simulink library "HardwareIO"  (R2017b)
settings: Solver=FixedStepDiscrete  StartTime=0.0  StopTime=inf  RelTol=1e-3  EnableMultiTasking=on
undefined symbols (not defined in the file or in its folder): Normalized
libraries: dspsrcs4 x1
settings Model: Creator=mcuenant  LastModifiedBy=mcuenant
settings DataIOCC: SaveFormat=Array  SaveOutput=off  SaveTime=off
settings OptimizationCC: LifeSpan=Inf
settings DebuggingCC: SFUnexpectedBacktrackingDiag=warning  SFNoUnconditionalDefaultTransitionDiag=warning  SFExecutionAtInitializationDiag=none
settings HardwareCC: ProdBitPerPointer=32  ProdBitPerSizeT=32  ProdBitPerPtrDiffT=32  ProdLargestAtomicFloat=None  ProdWordSize=32  ProdHWDeviceType=Generic->32-bit x86 compatible
settings ModelReferenceCC: PropagateSignalLabelsOutOfModel=off
settings SFSimCC: MATLABDynamicMemAlloc=off
settings RTWCC: SystemTargetFile=ert.tlc  GenCodeOnly=on  TemplateMakefile=ert_default_tmf  GenerateReport=on  IncludeHyperlinkInReport=on  LaunchReport=on  PortableWordSizes=on  CodeProfilingSaveOptions=AllData  GenerateTraceInfo=on  GenerateTraceReport=on  GenerateTraceReportSl=on  GenerateTraceReportSf=on  GenerateTraceReportEml=on  GenerateWebview=on  GenerateCodeMetricsReport=on  GenerateCodeReplacementReport=on
settings CodeAppCC: IgnoreCustomStorageClasses=off  MaxIdLength=128  SimulinkDataObjDesc=on  SFDataObjDesc=on  InsertBlockDesc=on  StateflowObjectComments=on  MATLABSourceComments=on  ReqsInCode=on
settings ERTTargetCC: MultiwordLength=2048  GenerateSampleERTMain=on  SupportAbsoluteTime=off  SupportNonFinite=off  SupportComplex=off  ERTCustomFileTemplate=example_file_process.tlc  ConvertIfToSwitch=off  SuppressUnreachableDefaultCases=off
settings ConfigComp: CovMetricSettings=dw  CovSaveCumulativeToWorkspaceVar=on  CovSaveSingleToWorkspaceVar=on  CovExternalEMLEnable=off

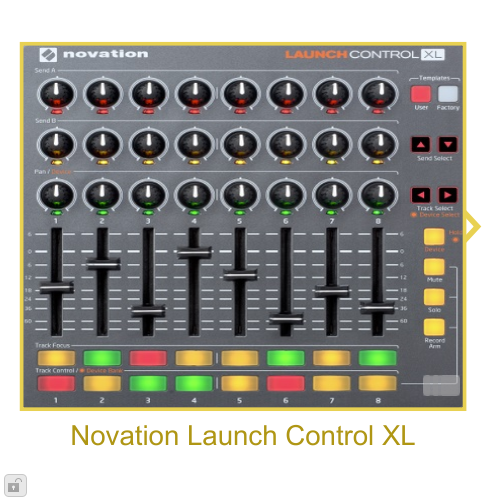
[thumbnail: Simulink's stored preview of the top-level diagram]
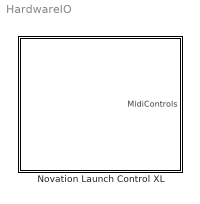
== system HardwareIO ==
  Novation Launch Control XL : Subsystem  TreatAsAtomicUnit=on  mask{Tso=0.1, Tsi=0.1, rtp=off, kA1=[0  1], kA2=[0  1], kA3=[0  1], kA4=[0  1], kA5=[0  1], kA6=[0  1], kA7=[0  1], kA8=[0  1], skA1=Linear, skA2=Linear, skA3=Linear, skA4=Linear, skA5=Linear, skA6=Linear, skA7=Linear, skA8=Linear, kB1=[0  1], kB2=[0  1], kB3=[0  1], kB4=[0  1], kB5=[0  1], kB6=[0  1], kB7=[0  1], kB8=[0  1], skB1=Linear, skB2=Linear, skB3=Linear, skB4=Linear, skB5=Linear, skB6=Linear, skB7=Linear, skB8=Linear, kC1=[0  1], kC2=[0  1], kC3=[0  1], kC4=[0  1], kC5=[0  1], kC6=[0  1], kC7=[0  1], kC8=[0  1], skC1=Linear, skC2=Linear, skC3=Linear, skC4=Linear, skC5=Linear, skC6=Linear, skC7=Linear, skC8=Linear, f1=[0  1], f2=[0  1], f3=[0  1], f4=[0  1], f5=[0  1], f6=[0  1], f7=[0  1], f8=[0  1], sf1=Linear, sf2=Linear, sf3=Linear, sf4=Linear, sf5=Linear, sf6=Linear, sf7=Linear, sf8=Linear}
      mask prompts: Tso "Output Sample Time (s)"; Tsi "Inner Sample Time for MIDI capture (s)   -   Recommended Value : 0.1 s"; rtp "Real-Time Pacer"; kA1 "Knob A1"; kA2 "Knob A2"; kA3 "Knob A3"; kA4 "Knob A4"; kA5 "Knob A5"; kA6 "Knob A6"; kA7 "Knob A7"; kA8 "Knob A8"; skA1 "Scale"; skA2 "Scale"; skA3 "Scale"; skA4 "Scale"; skA5 "Scale"; skA6 "Scale"; skA7 "Scale"; skA8 "Scale"; kB1 "Knob B1"; kB2 "Knob B2"; kB3 "Knob B3"; kB4 "Knob B4"; kB5 "Knob B5"; kB6 "Knob B6"; kB7 "Knob B7"; kB8 "Knob B8"; skB1 "Scale"; skB2 "Scale"; skB3 "Scale"; skB4 "Scale"; skB5 "Scale"; skB6 "Scale"; skB7 "Scale"; skB8 "Scale"; kC1 "Knob C1"; kC2 "Knob C2"; kC3 "Knob C3"; kC4 "Knob C4"; kC5 "Knob C5"; kC6 "Knob C6"; kC7 "Knob C7"; kC8 "Knob C8"; skC1 "Scale"; skC2 "Scale"; skC3 "Scale"; skC4 "Scale"; skC5 "Scale"; skC6 "Scale"; skC7 "Scale"; skC8 "Scale"; f1 "Fader F1"; f2 "Fader F2"; f3 "Fader F3"; f4 "Fader F4"; f5 "Fader F5"; f6 "Fader F6"; f7 "Fader F7"; f8 "Fader F8"; sf1 "Scale"; sf2 "Scale"; sf3 "Scale"; sf4 "Scale"; sf5 "Scale"; sf6 "Scale"; sf7 "Scale"; sf8 "Scale"
      mask init:
      | %% Parameters
      | maxIntervals = 20; % maximum number of values for N-ary mode
      | 
      | %% Generate cell with button names
      | knobsA = arrayfun(@(x) ['Knob A' num2str(x)],1:8,'UniformOutput',false);
      | knobsB = arrayfun(@(x) ['Knob B' num2str(x)],1:8,'UniformOutput',false);
      | knobsC = arrayfun(@(x) ['Knob C' num2str(x)],1:8,'UniformOutput',false);
      | faders = arrayfun(@(x) ['Fader F' num2str(x)],1:8,'UniformOutput',false);
      | buttons = [knobsA(:) ; knobsB(:) ; knobsC(:) ; faders(:)];
      | 
      | 
      | %% Gather parameters in an array of structures
      | param(1).value = kA1;
      | param(1).scale = skA1;
      | param(2).value = kA2;
      | param(2).scale = skA2;
      | param(3).value = kA3;
      | param(3).scale = skA3;
      | param(4).value = kA4;
      | param(4).scale = skA4;
      | param(5).value = kA5;
      | param(5).scale = skA5;
      | param(6).value = kA6;
      | param(6).scale = skA6;
      | param(7).value = kA7;
      | param(7).scale = skA7;
      | param(8).value = kA8;
      | param(8).scale = skA8;
      | param(9).value = kB1;
      | param(9).scale = skB1;
      | param(10).value = kB2;
      | param(10).scale = skB2;
      | param(11).value = kB3;
      | param(11).scale = skB3;
      | param(12).value = kB4;
      | param(12).scale = skB4;
      | param(13).value = kB5;
      | param(13).scale = skB5;
      | param(14).value = kB6;
      | param(14).scale = skB6;
      | param(15).value = kB7;
      | param(15).scale = skB7;
      | param(16).value = kB8;
      | param(16).scale = skB8;
      | param(17).value = kC1;
      | param(17).scale = skC1;
      | param(18).value = kC2;
      | param(18).scale = skC2;
      | param(19).value = kC3;
      | param(19).scale = skC3;
      | param(20).value = kC4;
      | param(20).scale = skC4;
      | param(21).value = kC5;
      | param(21).scale = skC5;
      | param(22).value = kC6;
      | param(22).scale = skC6;
      | param(23).value = kC7;
      | param(23).scale = skC7;
      | param(24).value = kC8;
      | param(24).scale = skC8;
      | param(25).value = f1;
      | param(25).scale = sf1;
      | param(26).value = f2;
      | param(26).scale = sf2;
      | param(27).value = f3;
      | param(27).scale = sf3;
      | param(28).value = f4;
      | param(28).scale = sf4;
      | param(29).value = f5;
      | param(29).scale = sf5;
      | param(30).value = f6;
      | param(30).scale = sf6;
      | param(31).value = f7;
      | param(31).scale = sf7;
      | param(32).value = f8;
      | param(32).scale = sf8;
      | 
      | %% Check User Inputs
      | funcName = 'Buttons parameters';
      | for ind=1:length(param)
      |     varName = buttons{ind};
      |     switch param(ind).scale
      |         case 1 % 'Linear'
      |             errMsgName = [varName, ' (using linear scale)'];
      |             validateattributes(param(ind).value,...
      |                 {'numeric'},{'increasing','finite','row','numel',2},...
      |                 funcName,errMsgName);
      |         case 2 % 'Logarithmic'
      |             errMsgName = [varName, ' (using log scale)'];
      |             validateattributes(param(ind).value,...
      |                 {'numeric'},{'increasing','finite','row','numel',2,'>',0},...
      |                 funcName,errMsgName);
      |         case 3 % 'Binary'
      |             errMsgName = [varName, ' (using N-ary scale)'];
      |             validateattributes(param(ind).value,...
      |                 {'numeric'},{'finite','row'},...
      |                 funcName,errMsgName);
      |             if (numel(param(ind).value) < 2 || numel(param(ind).value) > maxIntervals)
      |                 errordlg(['When using N-ary scaling, you must supply between 2 and ' num2str(maxIntervals) ' values to define intervals.'])
      |             end
      |     end
      | end
      | 
      | clear kA1 kA2 kA3 kA4 kA5 kA6 kA7 kA8 kB1 kB2 kB3 kB4 kB5 kB6 kB7 kB8 kC1 kC2 kC3 kC4 kC5 kC6 kC7 kC8 f1 f2 f3 f4 f5 f6 f7 f8 skA1 skA2 skA3 skA4 skA5 skA6 skA7 skA8 skB1 skB2 skB3 skB4 skB5 skB6 skB7 skB8 skC1 skC2 skC3 skC4 skC5 skC6 skC7 skC8 sf1 sf2 sf3 sf4 sf5 sf6 sf7 sf8;
      | clear knobsA knobsB knobsC faders buttons;
      | clear funcName varName errMsgName;
      | 
      | %% Pad with NaN to allow N-ary scale (field "value" of structure array param must have a consistent size across array elements)
      | param(1).value = [param(1).value, NaN(1,maxIntervals-length(param(1).value))];
      | param(2).value = [param(2).value, NaN(1,maxIntervals-length(param(2).value))];
      | param(3).value = [param(3).value, NaN(1,maxIntervals-length(param(3).value))];
      | param(4).value = [param(4).value, NaN(1,maxIntervals-length(param(4).value))];
      | param(5).value = [param(5).value, NaN(1,maxIntervals-length(param(5).value))];
      | param(6).value = [param(6).value, NaN(1,maxIntervals-length(param(6).value))];
      | param(7).value = [param(7).value, NaN(1,maxIntervals-length(param(7).value))];
      | param(8).value = [param(8).value, NaN(1,maxIntervals-length(param(8).value))];
      | param(9).value = [param(9).value, NaN(1,maxIntervals-length(param(9).value))];
      | param(10).value = [param(10).value, NaN(1,maxIntervals-length(param(10).value))];
      | param(11).value = [param(11).value, NaN(1,maxIntervals-length(param(11).value))];
      | param(12).value = [param(12).value, NaN(1,maxIntervals-length(param(12).value))];
      | param(13).value = [param(13).value, NaN(1,maxIntervals-length(param(13).value))];
      | param(14).value = [param(14).value, NaN(1,maxIntervals-length(param(14).value))];
      | param(15).value = [param(15).value, NaN(1,maxIntervals-length(param(15).value))];
      | param(16).value = [param(16).value, NaN(1,maxIntervals-length(param(16).value))];
      | param(17).value = [param(17).value, NaN(1,maxIntervals-length(param(17).value))];
      | param(18).value = [param(18).value, NaN(1,maxIntervals-length(param(18).value))];
      | param(19).value = [param(19).value, NaN(1,maxIntervals-length(param(19).value))];
      | param(20).value = [param(20).value, NaN(1,maxIntervals-length(param(20).value))];
      | param(21).value = [param(21).value, NaN(1,maxIntervals-length(param(21).value))];
      | param(22).value = [param(22).value, NaN(1,maxIntervals-length(param(22).value))];
      | param(23).value = [param(23).value, NaN(1,maxIntervals-length(param(23).value))];
      | param(24).value = [param(24).value, NaN(1,maxIntervals-length(param(24).value))];
      | param(25).value = [param(25).value, NaN(1,maxIntervals-length(param(25).value))];
      | param(26).value = [param(26).value, NaN(1,maxIntervals-length(param(26).value))];
      | param(27).value = [param(27).value, NaN(1,maxIntervals-length(param(27).value))];
      | param(28).value = [param(28).value, NaN(1,maxIntervals-length(param(28).value))];
      | param(29).value = [param(29).value, NaN(1,maxIntervals-length(param(29).value))];
      | param(30).value = [param(30).value, NaN(1,maxIntervals-length(param(30).value))];
      | param(31).value = [param(31).value, NaN(1,maxIntervals-length(param(31).value))];
      | param(32).value = [param(32).value, NaN(1,maxIntervals-length(param(32).value))];
      | clear maxIntervals;
      mask TypeOptions skA1: Linear | Logarithmic | N-ary
      mask TypeOptions skA2: Linear | Logarithmic | N-ary
      mask TypeOptions skA3: Linear | Logarithmic | N-ary
      mask TypeOptions skA4: Linear | Logarithmic | N-ary
      mask TypeOptions skA5: Linear | Logarithmic | N-ary
      mask TypeOptions skA6: Linear | Logarithmic | N-ary
      mask TypeOptions skA7: Linear | Logarithmic | N-ary
      mask TypeOptions skA8: Linear | Logarithmic | N-ary
      mask TypeOptions skB1: Linear | Logarithmic | N-ary
      mask TypeOptions skB2: Linear | Logarithmic | N-ary
      mask TypeOptions skB3: Linear | Logarithmic | N-ary
      mask TypeOptions skB4: Linear | Logarithmic | N-ary
      mask TypeOptions skB5: Linear | Logarithmic | N-ary
      mask TypeOptions skB6: Linear | Logarithmic | N-ary
      mask TypeOptions skB7: Linear | Logarithmic | N-ary
      mask TypeOptions skB8: Linear | Logarithmic | N-ary
      mask TypeOptions skC1: Linear | Logarithmic | N-ary
      mask TypeOptions skC2: Linear | Logarithmic | N-ary
      mask TypeOptions skC3: Linear | Logarithmic | N-ary
      mask TypeOptions skC4: Linear | Logarithmic | N-ary
      mask TypeOptions skC5: Linear | Logarithmic | N-ary
      mask TypeOptions skC6: Linear | Logarithmic | N-ary
      mask TypeOptions skC7: Linear | Logarithmic | N-ary
      mask TypeOptions skC8: Linear | Logarithmic | N-ary
      mask TypeOptions sf1: Linear | Logarithmic | N-ary
      mask TypeOptions sf2: Linear | Logarithmic | N-ary
      mask TypeOptions sf3: Linear | Logarithmic | N-ary
      mask TypeOptions sf4: Linear | Logarithmic | N-ary
      mask TypeOptions sf5: Linear | Logarithmic | N-ary
      mask TypeOptions sf6: Linear | Logarithmic | N-ary
      mask TypeOptions sf7: Linear | Logarithmic | N-ary
      mask TypeOptions sf8: Linear | Logarithmic | N-ary
      mask DialogControl DescGroupVar Prompt: Novation Launch Control XL
      mask DialogControl DescTextVar Prompt: Block for capturing inputs from MIDI console Novation Launch Control XL.
      mask DialogControl ParameterGroupVar Prompt: Sample times
      mask DialogControl Container11 Prompt: Knobs scaling [min  max]
      mask DialogControl Container5 Prompt: A set  [Send A]
      mask DialogControl Container6 Prompt: B set  [Send B]
      mask DialogControl Container8 Prompt: C set  [Pan / Device]
      mask DialogControl Container12 Prompt: Faders scaling [min  max]
      mask Display: image('LaunchControlXL.jpg')

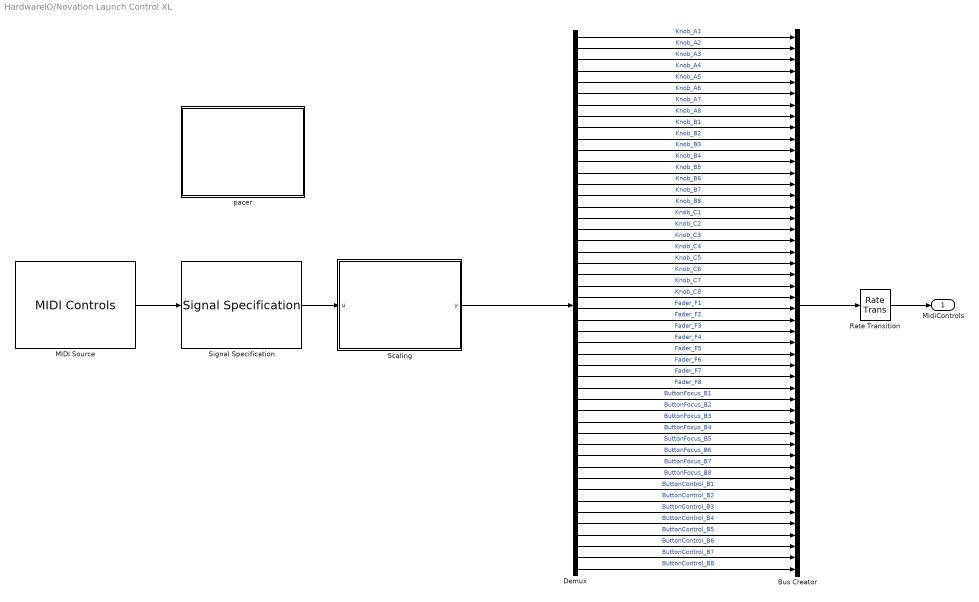
== system HardwareIO/Novation Launch Control XL ==
  Bus Creator : BusCreator  Inputs=48
  Demux : Demux  Outputs=48
  MIDI Source : dspsrcs4/MIDI Controls  UseSpecifiedDevice=Specify other  DeviceName='Launch Control XL'  UseSpecifiedControls=Respond to specified controls  ControlNumbers="[13:20  29:36  49:56  77:84  41:44 57:60  73:76 89:92]"  InitialValues=0  SyncAtStart=off  RawUint8=Normalized (0 - 1)
  Rate Transition : RateTransition  Integrity=off  Deterministic=off  OutPortSampleTime=Tso
  Scaling : MATLAB Function  TreatAsAtomicUnit=on
  Signal Specification : SignalSpecification  SampleTime=Tsi
  pacer : Subsystem  TreatAsAtomicUnit=on  mask{samp=Tsi, rate=rtp}
      mask prompts: samp "Sample time"; rate "Rate (2 = twice faster than real-time)"
      mask Display:
      | if rate > 0
      |     disp(['PACER\nx', num2str(rate)]);
      | else
      |     disp('PACER\nInactive');
      | end
  MidiControls : Outport  VectorParamsAs1DForOutWhenUnconnected=off
  wires:
  Scaling/1(y) -> Demux/1
  Rate Transition/1 -> MidiControls/1
  Demux/2 -> Bus Creator/2  "Knob_A2"
  Demux/19 -> Bus Creator/19  "Knob_C3"
  Demux/47 -> Bus Creator/47  "ButtonControl_B7"
  Demux/45 -> Bus Creator/45  "ButtonControl_B5"
  Demux/44 -> Bus Creator/44  "ButtonControl_B4"
  Demux/46 -> Bus Creator/46  "ButtonControl_B6"
  Demux/48 -> Bus Creator/48  "ButtonControl_B8"
  Demux/3 -> Bus Creator/3  "Knob_A3"
  Demux/14 -> Bus Creator/14  "Knob_B6"
  Demux/15 -> Bus Creator/15  "Knob_B7"
  Demux/12 -> Bus Creator/12  "Knob_B4"
  Demux/29 -> Bus Creator/29  "Fader_F5"
  Demux/30 -> Bus Creator/30  "Fader_F6"
  Demux/31 -> Bus Creator/31  "Fader_F7"
  Demux/32 -> Bus Creator/32  "Fader_F8"
  Demux/33 -> Bus Creator/33  "ButtonFocus_B1"
  Demux/34 -> Bus Creator/34  "ButtonFocus_B2"
  Demux/35 -> Bus Creator/35  "ButtonFocus_B3"
  Demux/36 -> Bus Creator/36  "ButtonFocus_B4"
  Demux/37 -> Bus Creator/37  "ButtonFocus_B5"
  Demux/38 -> Bus Creator/38  "ButtonFocus_B6"
  Demux/39 -> Bus Creator/39  "ButtonFocus_B7"
  Demux/40 -> Bus Creator/40  "ButtonFocus_B8"
  Demux/41 -> Bus Creator/41  "ButtonControl_B1"
  Demux/42 -> Bus Creator/42  "ButtonControl_B2"
  Demux/43 -> Bus Creator/43  "ButtonControl_B3"
  Demux/22 -> Bus Creator/22  "Knob_C6"
  Demux/26 -> Bus Creator/26  "Fader_F2"
  Demux/7 -> Bus Creator/7  "Knob_A7"
  Demux/1 -> Bus Creator/1  "Knob_A1"
  Demux/5 -> Bus Creator/5  "Knob_A5"
  Demux/21 -> Bus Creator/21  "Knob_C5"
  Demux/13 -> Bus Creator/13  "Knob_B5"
  Demux/9 -> Bus Creator/9  "Knob_B1"
  Demux/4 -> Bus Creator/4  "Knob_A4"
  Demux/27 -> Bus Creator/27  "Fader_F3"
  Demux/24 -> Bus Creator/24  "Knob_C8"
  Demux/20 -> Bus Creator/20  "Knob_C4"
  Demux/23 -> Bus Creator/23  "Knob_C7"
  Demux/18 -> Bus Creator/18  "Knob_C2"
  Demux/28 -> Bus Creator/28  "Fader_F4"
  Demux/25 -> Bus Creator/25  "Fader_F1"
  Demux/10 -> Bus Creator/10  "Knob_B2"
  Demux/17 -> Bus Creator/17  "Knob_C1"
  Demux/6 -> Bus Creator/6  "Knob_A6"
  Demux/16 -> Bus Creator/16  "Knob_B8"
  Demux/8 -> Bus Creator/8  "Knob_A8"
  Demux/11 -> Bus Creator/11  "Knob_B3"
  Signal Specification/1 -> Scaling/1(u)
  Bus Creator/1 -> Rate Transition/1
  MIDI Source/1 -> Signal Specification/1

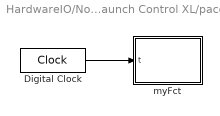
== system HardwareIO/Novation Launch Control XL/pacer ==
  Digital Clock : DigitalClock  SampleTime=samp
  myFct : MATLAB Function  TreatAsAtomicUnit=on
  wires:
  Digital Clock/1 -> myFct/1(t)

== matlab function HardwareIO/Novation Launch Control XL/Scaling ==
  data: u input; y output; param parameter
function y = fcn(u,param)
%#codegen

% Pre-allocation
y = u;

% Knobs and faders scaling (index 1 to 32)
for ind=1:length(param)
    switch param(ind).scale
        case 1 % 'Linear'
            a = param(ind).value(2)-param(ind).value(1);
            b = param(ind).value(1);
            y(ind) = a*u(ind)+b;
            
        case 2 % 'Logarithmic'
            a = param(ind).value(1);
            b = param(ind).value(2)/param(ind).value(1);
            y(ind) = a*b.^u(ind);
            
        case 3 % 'N-ary' : use supplied values without interpolation (hard switching)
            N = sum(~isnan(param(ind).value));
            idx = min(1+floor(u(ind)*N),N);
            y(ind) = param(ind).value(idx);
    end
end

== matlab function HardwareIO/Novation Launch Control XL/pacer/myFct ==
  data: t input; rate parameter size=1
function fcn(t, rate)
%#codegen

% Coder
coder.extrinsic('clock', 'etime')

% Activation / deactivation
if rate <= 0
    return
end

% Persistent variable
persistent t0

if isempty(t0)
	t0 = clock;
	return;
end

% Pacer
y = 0;
y = etime(clock, t0);
while y < (t/rate)
	y = etime(clock, t0);
end
